simulink subsystem "Aerodynamics"  (R2021b)
settings: Solver=VariableStepAuto  StartTime=0.0  StopTime=10.0  RelTol=1e-3
values from neighbouring files (symbols this model uses):
  R = zeros(3)    [eul2rotmat.m]
undefined symbols (not defined in the file or in its folder): aircraft, CD_tether, S_tether, wing1
libraries: aerolibasang x2, aerolibadyn x1
settings Model: Creator=austm  LastModifiedBy=austm

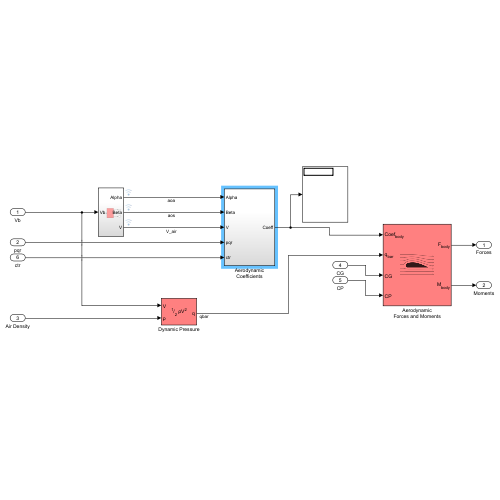
[thumbnail: Simulink's stored preview of the top-level diagram]
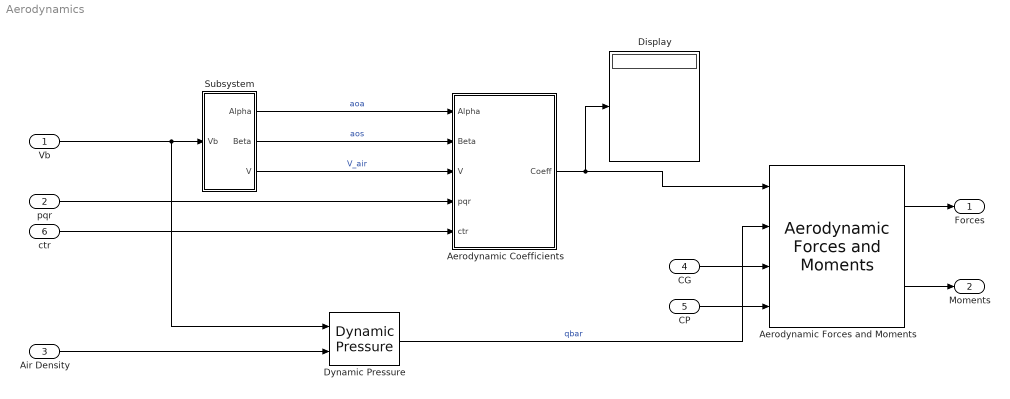
== system Aerodynamics ==
  Vb : Inport
  pqr : Inport  Port=2
  Air Density : Inport  Port=3
  CG : Inport  Port=4
  CP : Inport  Port=5
  ctr : Inport  Port=6
  Aerodynamic Coefficients : Subsystem
  Aerodynamic Forces and Moments : aerolibadyn/Aerodynamic Forces and Moments   inputAxes=Body  outputForceAxes=Body  outputMomentAxes=Body  S=wing1.ReferenceArea  b=wing1.ReferenceSpan  cbar=wing1.ReferenceLength
  Display : Display
  Dynamic Pressure : aerolibasang/Dynamic Pressure
  Subsystem : Subsystem
  Forces : Outport
  Moments : Outport  Port=2
  wires:
  Dynamic Pressure/1 -> Aerodynamic Forces and Moments/2  "qbar"
  Vb/1 -> Dynamic Pressure/1, Subsystem/1(Vb)
  Subsystem/2(Beta) -> Aerodynamic Coefficients/2(Beta)  "aos"
  CP/1 -> Aerodynamic Forces and Moments/4
  Subsystem/3(V) -> Aerodynamic Coefficients/3(V)  "V_air"
  Subsystem/1(Alpha) -> Aerodynamic Coefficients/1(Alpha)  "aoa"
  Aerodynamic Coefficients/1(Coeff) -> Aerodynamic Forces and Moments/1, Display/1
  CG/1 -> Aerodynamic Forces and Moments/3
  Air Density/1 -> Dynamic Pressure/2
  Aerodynamic Forces and Moments/2 -> Moments/1
  Aerodynamic Forces and Moments/1 -> Forces/1
  pqr/1 -> Aerodynamic Coefficients/4(pqr)
  ctr/1 -> Aerodynamic Coefficients/5(ctr)

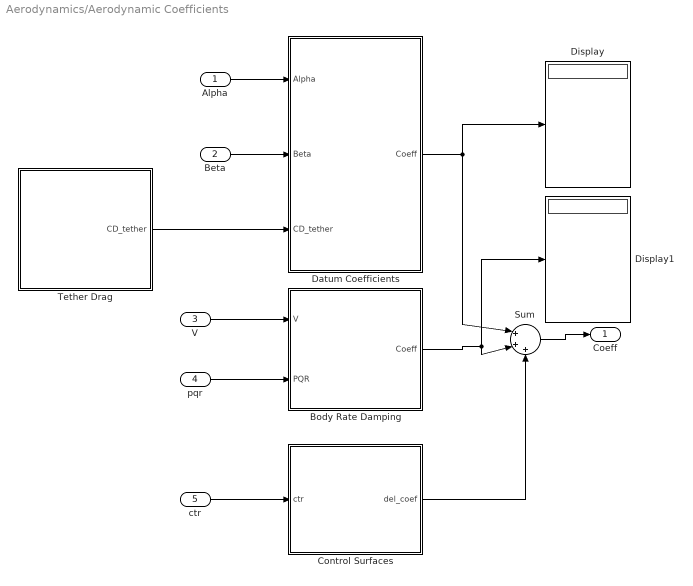
== system Aerodynamics/Aerodynamic Coefficients ==
  Alpha : Inport
  Beta : Inport  Port=2
  V : Inport  Port=3
  pqr : Inport  Port=4  Unit=m/s
  ctr : Inport  Port=5
  Body Rate Damping : Subsystem
  Control Surfaces : Subsystem
  Datum Coefficients : Subsystem
  Display : Display
  Display1 : Display
  Sum : Sum  Inputs=|+++
  Tether Drag : Subsystem
  Coeff : Outport  VectorParamsAs1DForOutWhenUnconnected=off
  wires:
  Control Surfaces/1(del_coef) -> Sum/3
  ctr/1 -> Control Surfaces/1(ctr)
  pqr/1 -> Body Rate Damping/2(PQR)
  Body Rate Damping/1(Coeff) -> Display1/1, Sum/2
  Alpha/1 -> Datum Coefficients/1(Alpha)
  Beta/1 -> Datum Coefficients/2(Beta)
  Datum Coefficients/1(Coeff) -> Sum/1, Display/1
  V/1 -> Body Rate Damping/1(V)
  Sum/1 -> Coeff/1
  Tether Drag/1(CD_tether) -> Datum Coefficients/3(CD_tether)

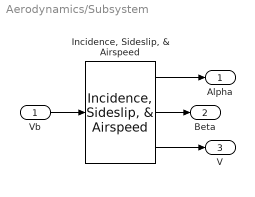
== system Aerodynamics/Subsystem ==
  Vb : Inport
  "Incidence, Sideslip, & Airspeed" : aerolibasang/Incidence, Sideslip, & Airspeed
  Alpha : Outport
  Beta : Outport  Port=2
  V : Outport  Port=3
  wires:
  "Incidence, Sideslip, & Airspeed"/2 -> Beta/1
  "Incidence, Sideslip, & Airspeed"/1 -> Alpha/1
  Vb/1 -> "Incidence, Sideslip, & Airspeed"/1
  "Incidence, Sideslip, & Airspeed"/3 -> V/1

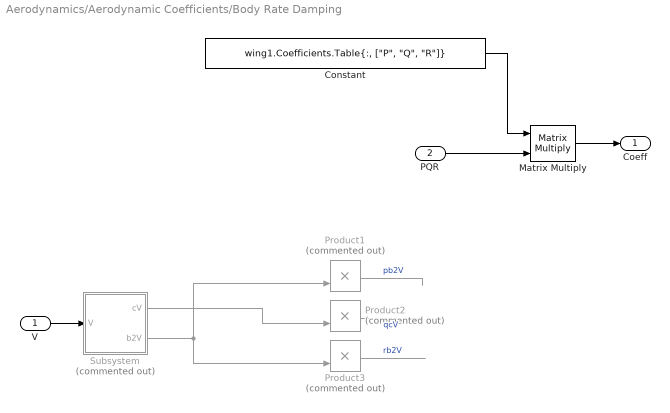
== system Aerodynamics/Aerodynamic Coefficients/Body Rate Damping ==
  V : Inport  Unit=m/s
  PQR : Inport  Port=2
  Constant : Constant  Value="wing1.Coefficients.Table{:, [\"P\", \"Q\", \"R\"]}"
  Matrix Multiply : Product  Multiplication=Matrix(*)
  Product1 : Product  Commented=on
  Product2 : Product  Commented=on
  Product3 : Product  Commented=on
  Subsystem : Subsystem  Commented=on
  Coeff : Outport  InitialOutput=0  VectorParamsAs1DForOutWhenUnconnected=off
  wires:
  V/1 -> Subsystem/1(V)
  Subsystem/1(cV) -> Product2/2
  Constant/1 -> Matrix Multiply/1
  Product3/1 -> ?  "rb2V"
  Subsystem/2(b2V) -> Product3/2, Product1/2
  Product2/1 -> ?  "qcV"
  Product1/1 -> ?  "pb2V"
  PQR/1 -> Matrix Multiply/2
  Matrix Multiply/1 -> Coeff/1

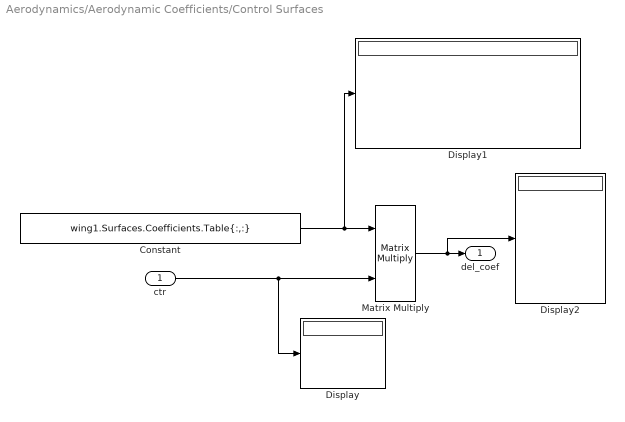
== system Aerodynamics/Aerodynamic Coefficients/Control Surfaces ==
  ctr : Inport
  Constant : Constant  Value=wing1.Surfaces.Coefficients.Table{:,:}
  Display : Display
  Display1 : Display
  Display2 : Display
  Matrix Multiply : Product  Multiplication=Matrix(*)
  del_coef : Outport
  wires:
  Matrix Multiply/1 -> del_coef/1, Display2/1
  ctr/1 -> Matrix Multiply/2, Display/1
  Constant/1 -> Matrix Multiply/1, Display1/1

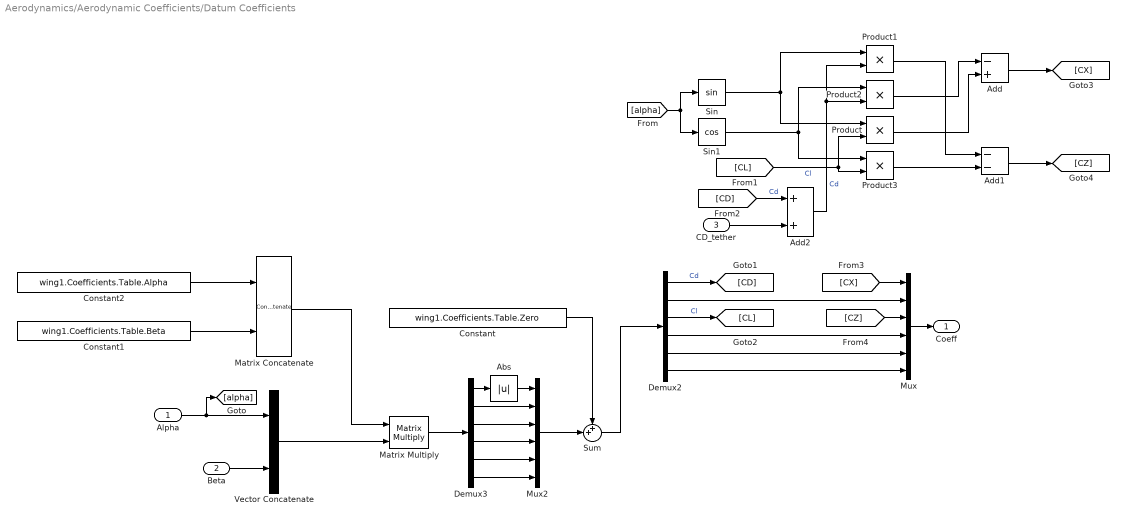
== system Aerodynamics/Aerodynamic Coefficients/Datum Coefficients ==
  Alpha : Inport
  Beta : Inport  Port=2
  CD_tether : Inport  Port=3
  Abs : Abs
  Add : Sum  Inputs=-+
  Add1 : Sum  Inputs=--
  Add2 : Sum
  Constant : Constant  Value=wing1.Coefficients.Table.Zero
  Constant1 : Constant  Value=wing1.Coefficients.Table.Beta
  Constant2 : Constant  Value=wing1.Coefficients.Table.Alpha
  Demux2 : Demux  Outputs=6
  Demux3 : Demux  Outputs=6
  Matrix Concatenate : Concatenate  Mode=Multidimensional array  ConcatenateDimension=2
  Matrix Multiply : Product  Multiplication=Matrix(*)
  Mux : Mux  Inputs=6
  Mux2 : Mux  Inputs=6
  Product{,1..3} (4 alike) : Product
  Sin : Trigonometry
  Sin1 : Trigonometry  Operator=cos
  Sum : Sum  Inputs=++|
  Vector Concatenate : Concatenate
  Coeff : Outport  InitialOutput=0  VectorParamsAs1DForOutWhenUnconnected=off
  wires:
  Matrix Concatenate/1 -> Matrix Multiply/1
  Abs/1 -> Mux2/1
  Mux2/1 -> Sum/2
  Demux3/1 -> Abs/1
  Demux3/4 -> Mux2/4
  Demux3/3 -> Mux2/3
  Demux3/2 -> Mux2/2
  Demux3/5 -> Mux2/5
  Demux3/6 -> Mux2/6
  [CL] -> Product/2, Product3/2  "Cl"
  Demux2/2 -> Mux/2
  Add2/1 -> Product1/2, Product2/2  "Cd"
  Demux2/4 -> Mux/4
  Demux2/5 -> Mux/5
  Demux2/6 -> Mux/6
  Constant1/1 -> Matrix Concatenate/2
  Constant2/1 -> Matrix Concatenate/1
  Constant/1 -> Sum/1
  Beta/1 -> Vector Concatenate/2
  Vector Concatenate/1 -> Matrix Multiply/2
  Alpha/1 -> [alpha], Vector Concatenate/1
  Matrix Multiply/1 -> Demux3/1
  Sum/1 -> Demux2/1
  [alpha] -> Sin1/1, Sin/1
  Mux/1 -> Coeff/1
  Sin1/1 -> Product3/1, Product2/1
  Sin/1 -> Product/1, Product1/1
  Product3/1 -> Add1/2
  Product1/1 -> Add1/1
  Product/1 -> Add/2
  Product2/1 -> Add/1
  Add1/1 -> [CZ]
  Add/1 -> [CX]
  Demux2/3 -> [CL]  "Cl"
  Demux2/1 -> [CD]  "Cd"
  [CD] -> Add2/1  "Cd"
  CD_tether/1 -> Add2/2
  [CX] -> Mux/1
  [CZ] -> Mux/3

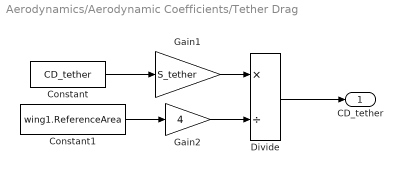
== system Aerodynamics/Aerodynamic Coefficients/Tether Drag ==
  Constant : Constant  Value=CD_tether
  Constant1 : Constant  Value=wing1.ReferenceArea
  Divide : Product  Inputs=*/
  Gain1 : Gain  Gain=S_tether
  Gain2 : Gain  Gain=4
  CD_tether : Outport
  wires:
  Constant/1 -> Gain1/1
  Constant1/1 -> Gain2/1
  Gain1/1 -> Divide/1
  Gain2/1 -> Divide/2
  Divide/1 -> CD_tether/1

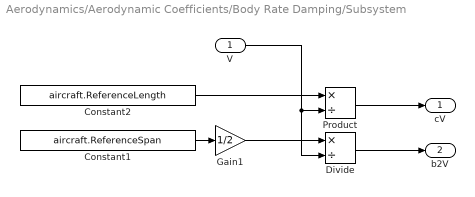
== system Aerodynamics/Aerodynamic Coefficients/Body Rate Damping/Subsystem ==
  V : Inport
  Constant1 : Constant  Value=aircraft.ReferenceSpan
  Constant2 : Constant  Value=aircraft.ReferenceLength
  Divide : Product  Inputs=*/
  Gain1 : Gain  Gain=1/2
  Product : Product  Inputs=*/
  cV : Outport
  b2V : Outport  Port=2
  wires:
  Gain1/1 -> Divide/1
  Constant2/1 -> Product/1
  Divide/1 -> b2V/1
  V/1 -> Product/2, Divide/2
  Constant1/1 -> Gain1/1
  Product/1 -> cV/1
